simulink model "offset_rate210_20160809_150859"  (R2014a)
settings: Solver=FixedStepDiscrete  SolverMode=SingleTasking  StartTime=0.0  StopTime=10.0  FixedStep=0.002  RelTol=1e-3
settings Model: BufferReuse=off  Creator=yoshi12  LastModifiedBy=yoshi12
settings OptimizationCC: BlockReduction=off  OptimizeBlockIOStorage=off  BufferReuse=off  GlobalBufferReuse=off  ExpressionFolding=off  LocalBlockOutputs=off  OptimizeModelRefInitCode=on  LifeSpan=1  SimCompilerOptimization=off
settings DebuggingCC: MergeDetectMultiDrivingBlocksExec=error  MultiTaskRateTransMsg=warning  FrameProcessingCompatibilityMsg=error
settings RTWCC: SystemTargetFile=ert.tlc  GenCodeOnly=on  TemplateMakefile=ert_default_tmf  Description=Embedded Coder  GenerateReport=on  IncludeHyperlinkInReport=on  LaunchReport=on  GenerateTraceInfo=on  GenerateTraceReport=on  GenerateTraceReportSl=on  GenerateTraceReportSf=on  GenerateTraceReportEml=on  RTWCompilerOptimization=off
settings CodeAppCC: IgnoreCustomStorageClasses=off
settings ERTTargetCC: ParMdlRefBuildCompliant=on  CompOptLevelCompliant=on  ConcurrentExecutionCompliant=on  ERTFirstTimeCompliant=on  ModelStepFunctionPrototypeControlCompliant=on  CPPClassGenCompliant=on  InlinedParameterPlacement=Hierarchical  ERTCustomFileTemplate=example_file_process.tlc
settings ConfigComp: CovMetricSettings=dw  CovHtmlReporting=on  CovSaveCumulativeToWorkspaceVar=on  CovSaveSingleToWorkspaceVar=on  CovModelRefEnable=Off  CovExternalEMLEnable=off  CovSFcnEnable=off

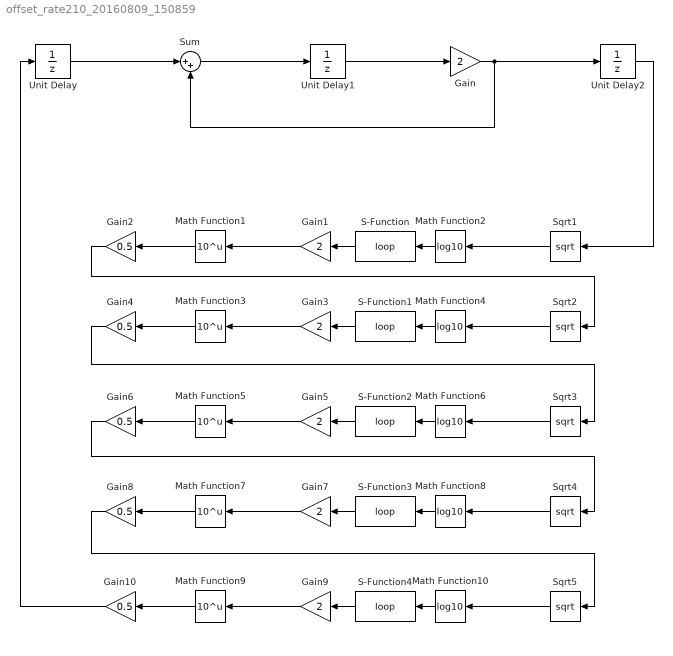
== system offset_rate210_20160809_150859 ==
  Gain : Gain  Gain=2  SampleTime=0.002
  Gain1 : Gain  Gain=2  SampleTime=[0.002,0]
  Gain10 : Gain  Gain=0.5  SampleTime=[0.01,0.008]
  Gain2 : Gain  Gain=0.5  SampleTime=[0.002,0]
  Gain3 : Gain  Gain=2  SampleTime=[0.004,0.002]
  Gain4 : Gain  Gain=0.5  SampleTime=[0.004,0.002]
  Gain5 : Gain  Gain=2  SampleTime=[0.006,0.004]
  Gain6 : Gain  Gain=0.5  SampleTime=[0.006,0.004]
  Gain7 : Gain  Gain=2  SampleTime=[0.008,0.006]
  Gain8 : Gain  Gain=0.5  SampleTime=[0.008,0.006]
  Gain9 : Gain  Gain=2  SampleTime=[0.01,0.008]
  Math Function1 : Math  Operator=10^u  SampleTime=[0.002,0]  SaturateOnIntegerOverflow=on
  Math Function10 : Math  Operator=log10  SampleTime=[0.01,0.008]  SaturateOnIntegerOverflow=on
  Math Function2 : Math  Operator=log10  SampleTime=[0.002,0]  SaturateOnIntegerOverflow=on
  Math Function3 : Math  Operator=10^u  SampleTime=[0.004,0.002]  SaturateOnIntegerOverflow=on
  Math Function4 : Math  Operator=log10  SampleTime=[0.004,0.002]  SaturateOnIntegerOverflow=on
  Math Function5 : Math  Operator=10^u  SampleTime=[0.006,0.004]  SaturateOnIntegerOverflow=on
  Math Function6 : Math  Operator=log10  SampleTime=[0.006,0.004]  SaturateOnIntegerOverflow=on
  Math Function7 : Math  Operator=10^u  SampleTime=[0.008,0.006]  SaturateOnIntegerOverflow=on
  Math Function8 : Math  Operator=log10  SampleTime=[0.008,0.006]  SaturateOnIntegerOverflow=on
  Math Function9 : Math  Operator=10^u  SampleTime=[0.01,0.008]  SaturateOnIntegerOverflow=on
  S-Function{,1..4} (5 alike) : S-Function  FunctionName=loop  EnableBusSupport=off
  Sqrt1 : Sqrt  SampleTime=[0.002,0]  SaturateOnIntegerOverflow=on
  Sqrt2 : Sqrt  SampleTime=[0.004,0.002]  SaturateOnIntegerOverflow=on
  Sqrt3 : Sqrt  SampleTime=[0.006,0.004]  SaturateOnIntegerOverflow=on
  Sqrt4 : Sqrt  SampleTime=[0.008,0.006]  SaturateOnIntegerOverflow=on
  Sqrt5 : Sqrt  SampleTime=[0.01,0.008]  SaturateOnIntegerOverflow=on
  Sum : Sum  Inputs=|++  SampleTime=0.002
  Unit Delay : UnitDelay  InitialCondition=1  SampleTime=-1
  Unit Delay1 : UnitDelay  InitialCondition=2  SampleTime=-1
  Unit Delay2 : UnitDelay  InitialCondition=1  SampleTime=-1
  wires:
  Unit Delay/1 -> Sum/1
  Sum/1 -> Unit Delay1/1
  Unit Delay1/1 -> Gain/1
  Gain/1 -> Sum/2, Unit Delay2/1
  Unit Delay2/1 -> Sqrt1/1
  Math Function3/1 -> Gain4/1
  Gain3/1 -> Math Function3/1
  Math Function4/1 -> S-Function1/1
  Sqrt2/1 -> Math Function4/1
  Math Function5/1 -> Gain6/1
  Gain5/1 -> Math Function5/1
  Math Function6/1 -> S-Function2/1
  Sqrt3/1 -> Math Function6/1
  Math Function7/1 -> Gain8/1
  Gain7/1 -> Math Function7/1
  Math Function8/1 -> S-Function3/1
  Sqrt4/1 -> Math Function8/1
  Math Function9/1 -> Gain10/1
  Gain9/1 -> Math Function9/1
  Math Function10/1 -> S-Function4/1
  Sqrt5/1 -> Math Function10/1
  Math Function1/1 -> Gain2/1
  Sqrt1/1 -> Math Function2/1
  Math Function2/1 -> S-Function/1
  Gain1/1 -> Math Function1/1
  Gain10/1 -> Unit Delay/1
  Gain2/1 -> Sqrt2/1
  Gain4/1 -> Sqrt3/1
  Gain6/1 -> Sqrt4/1
  Gain8/1 -> Sqrt5/1
  S-Function/1 -> Gain1/1
  S-Function1/1 -> Gain3/1
  S-Function2/1 -> Gain5/1
  S-Function3/1 -> Gain7/1
  S-Function4/1 -> Gain9/1
